simulink model "separator2020b"  (R2019a)
settings: Solver=VariableStepAuto  StartTime=0.0  StopTime=100  RelTol=1e-3
settings Model: Creator=amah2  LastModifiedBy=amah2

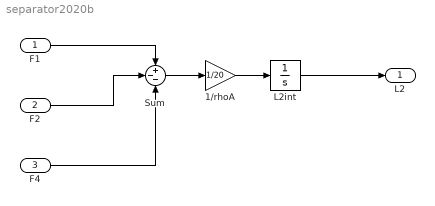
== system separator2020b ==
  F1 : Inport
  F2 : Inport  Port=2
  "F4 " : Inport  Port=3
  "1/rhoA " : Gain  Gain=1/20
  "L2int " : Integrator
  Sum : Sum  Inputs=+--
  L2 : Outport
  wires:
  F1/1 -> Sum/1
  F2/1 -> Sum/2
  "F4 "/1 -> Sum/3
  Sum/1 -> "1/rhoA "/1
  "1/rhoA "/1 -> "L2int "/1
  "L2int "/1 -> L2/1
